simulink model "fig5_32"  (Simulink 7.1)
settings: Solver=ode45  SolverMode=SingleTasking  StartTime=0.0  StopTime=2  RelTol=1e-3  AbsTol=1e-6
libraries: simulink x2
settings Model: Creator=Office Depot  LastModifiedBy=Office Depot  ExtModeTrigMode=oneshot  ExtModeArmWhenConnect=off
settings DataIOCC: LimitDataPoints=off
settings OptimizationCC: BlockReduction=off  BooleanDataType=off
settings DebuggingCC: SaveWithParameterizedLinksMsg=none  SignalResolutionControl=TryResolveAllWithWarning  SolverPrmCheckMsg=none  MultiTaskDSMMsg=warning  MultiTaskCondExecSysMsg=none  StrictBusMsg=None
settings HardwareCC: TargetUnknown=on
settings RTWCC: IncludeERTFirstTime=on
settings STFCustomTargetCC: ModelReferenceCompliant=off  SystemTargetFile=grt.tlc

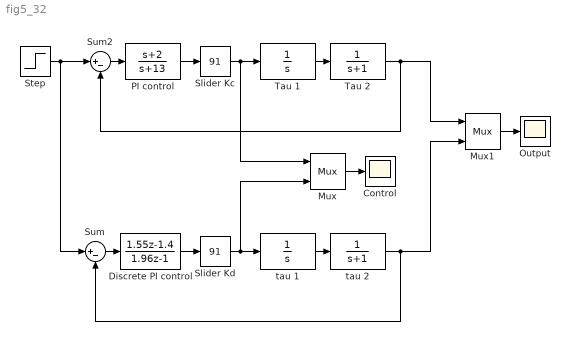
== system fig5_32 ==
  Control : Scope
      settings: TickLabels=on  YMin=0  YMax=2.75  SaveName=ucd  DataFormat=Array
  Discrete PI control : DiscreteTransferFcn  Numerator=[1.55 -1.4]  Denominator=[1.96 -1]  SampleTime=.05
  Mux : Mux  Inputs=2
  Mux1 : Mux  Inputs=2
  Output : Scope
      settings: TickLabels=on  SaveName=ycd  DataFormat=Array
  PI control : TransferFcn  Numerator="[1  2]"  Denominator=[1 13]
  Slider Kc : simulink/Math Operations/Slider Gain  SystemSampleTime=-1  low=0  gain=91  high=200
  Slider Kd : simulink/Math Operations/Slider Gain  SystemSampleTime=-1  low=0  gain=91  high=200
  Step : Step  Time=.1  SampleTime=.001
  Sum : Sum  Inputs=|+-  InputSameDT=on  OutDataTypeStr=Inherit: Same as first input
  Sum2 : Sum  Inputs=|+-  InputSameDT=on  OutDataTypeStr=Inherit: Same as first input
  Tau 1 : TransferFcn  Denominator=[1 0]
  Tau 2 : TransferFcn  Denominator=[1 1]
  tau 1 : TransferFcn  Denominator=[1 0]
  tau 2 : TransferFcn  Denominator=[1 1]
  wires:
  PI control/1 -> Slider Kc/1
  Sum2/1 -> PI control/1
  Tau 1/1 -> Tau 2/1
  Discrete PI control/1 -> Slider Kd/1
  tau 1/1 -> tau 2/1
  Step/1 -> Sum2/1, Sum/1
  Slider Kc/1 -> Tau 1/1, Mux/1
  Mux/1 -> Control/1
  Tau 2/1 -> Mux1/1, Sum2/2
  Mux1/1 -> Output/1
  Sum/1 -> Discrete PI control/1
  Slider Kd/1 -> tau 1/1, Mux/2
  tau 2/1 -> Mux1/2, Sum/2
